simulink library "I2C_SP"  (R2016b)
settings: Solver=VariableStepAuto  StartTime=0.0  StopTime=10.0  RelTol=1e-3
settings Model: Creator=taylorreynolds  LastModifiedBy=taylorreynolds

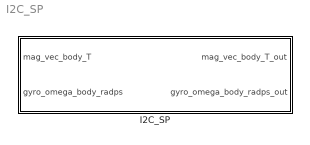
== system I2C_SP ==
  I2C_SP : Subsystem

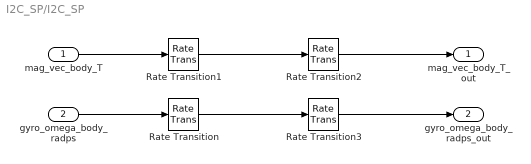
== system I2C_SP/I2C_SP ==
  mag_vec_body_T : Inport
  gyro_omega_body_radps : Inport  Port=2
  Rate Transition : RateTransition  OutPortSampleTime=sim_params.sensors.gyro.sample_time_s
  Rate Transition1 : RateTransition  OutPortSampleTime=sim_params.sensors.magnetometer.sample_time_s
  Rate Transition2 : RateTransition
  Rate Transition3 : RateTransition
  mag_vec_body_T_out : Outport
  gyro_omega_body_radps_out : Outport  Port=2
  wires:
  gyro_omega_body_radps/1 -> Rate Transition/1
  mag_vec_body_T/1 -> Rate Transition1/1
  Rate Transition1/1 -> Rate Transition2/1
  Rate Transition2/1 -> mag_vec_body_T_out/1
  Rate Transition/1 -> Rate Transition3/1
  Rate Transition3/1 -> gyro_omega_body_radps_out/1
